simulink model "ar03_sim_RST"  (R2020a)
settings: Solver=ode45  StartTime=0.0  StopTime=38  RelTol=1e-3  EnableMultiTasking=on
values from neighbouring files (symbols this model uses):
  A = [1 0.3 0.2]    [ar03_spustima_RMNS.m]    (also in ar03_spustima_STR.m)
  B = [0 0.15]    [ar03_spustima_RMNS.m]    (also in ar03_spustima_STR.m)
  Tvz = 0.1    [ar03_spustima_RMNS.m]    (also in ar03_spustima_STR.m)
settings Model: Creator=MT  LastModifiedBy=MT
settings DataIOCC: LimitDataPoints=on  SaveFormat=Array  SignalLoggingSaveFormat=ModelDataLogs  SaveOutput=off  SignalLogging=off  SaveTime=off  ReturnWorkspaceOutputs=off
settings OptimizationCC: ExpressionDepthLimit=2147483647  InitFltsAndDblsToZero=on  LifeSpan=inf
settings DebuggingCC: SaveWithParameterizedLinksMsg=none  UnderspecifiedInitializationDetection=Classic  MergeDetectMultiDrivingBlocksExec=none  SignalResolutionControl=TryResolveAllWithWarning  SolverPrmCheckMsg=warning  MultiTaskDSMMsg=warning  MultiTaskCondExecSysMsg=none  FcnCallInpInsideContextMsg=warning  AllowSymbolicDim=off  StateNameClashWarn=warning  SFUnexpectedBacktrackingDiag=warning  SFNoUnconditionalDefaultTransitionDiag=warning  SFExecutionAtInitializationDiag=none  ArithmeticOperatorsInVariantConditions=warning
settings HardwareCC: ProdBitPerPointer=32  ProdBitPerSizeT=32  ProdBitPerPtrDiffT=32  ProdLargestAtomicFloat=None  ProdIntDivRoundTo=Undefined  ProdEndianess=Unspecified  ProdWordSize=32  ProdHWDeviceType=32-bit Generic
settings ModelReferenceCC: PropagateSignalLabelsOutOfModel=off
settings SFSimCC: SimUseLocalCustomCode=off  CustomCodeUndefinedFunction=UseInterfaceOnly
settings RTWCC: RTWUseLocalCustomCode=off
settings CodeAppCC: StateflowObjectComments=on
settings GRTTargetCC: TargetFcnLib=ansi_tfl_tmw.mat  TargetLangStandard=C89/C90 (ANSI)  CombineOutputUpdateFcns=off  GRTInterface=on
settings ConfigComp: CovMetricSettings=dw  CovHtmlReporting=on  CovSaveCumulativeToWorkspaceVar=on  CovSaveSingleToWorkspaceVar=on  CovExternalEMLEnable=off

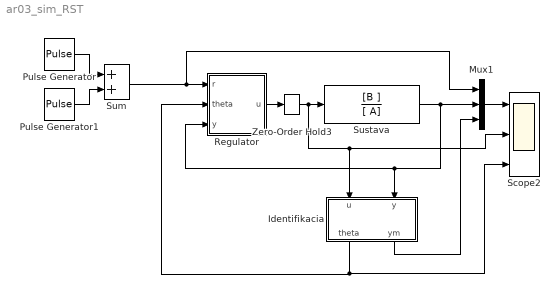
== system ar03_sim_RST ==
  Identifikacia : Subsystem
  Mux1 : Mux  Inputs=3
  Pulse Generator : DiscretePulseGenerator  PulseType=Time based  Period=40  PulseWidth=25
  Pulse Generator1 : DiscretePulseGenerator  PulseType=Time based  Amplitude=-1  Period=40  PulseWidth=25  PhaseDelay=20
  Regulator : Subsystem
  Scope2 : Scope  NumInputPorts=3
  Sum : Sum
  Sustava : TransferFcn  Numerator=[B ]  Denominator=[ A]
  Zero-Order Hold3 : ZeroOrderHold  SampleTime=Tvz
  wires:
  Sustava/1 -> Regulator/3(y), Identifikacia/2(y), Mux1/2
  Identifikacia/1(theta) -> Scope2/3, Regulator/2(theta)
  Mux1/1 -> Scope2/1
  Regulator/1(u) -> Zero-Order Hold3/1
  Zero-Order Hold3/1 -> Scope2/2, Identifikacia/1(u), Sustava/1
  Identifikacia/2(ym) -> Mux1/3
  Pulse Generator/1 -> Sum/1
  Pulse Generator1/1 -> Sum/2
  Sum/1 -> Mux1/1, Regulator/1(r)

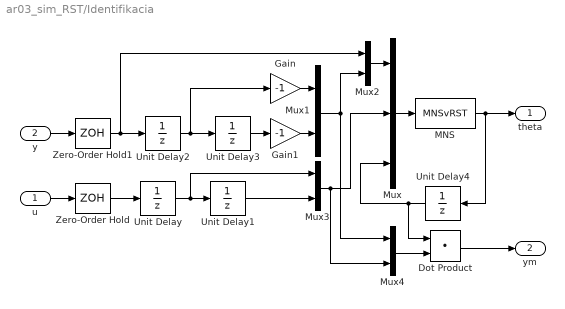
== system ar03_sim_RST/Identifikacia ==
  u : Inport
  y : Inport  Port=2
  Dot Product : DotProduct  InputSameDT=on  OutDataTypeStr=Inherit: Inherit via internal rule
  Gain : Gain  Gain=-1
  Gain1 : Gain  Gain=-1
  MNS : MATLABFcn  MATLABFcn=MNSvRST  OutputDimensions=4
  Mux : Mux  Inputs=3
  Mux{1..4} (4 alike) : Mux  Inputs=2
  Unit Delay{,1..3} (4 alike) : UnitDelay  SampleTime=Tvz  HasFrameUpgradeWarning=on
  Unit Delay4 : UnitDelay  InitialCondition="[-1.5    0.5    -2e-5    1.5e-3]"  SampleTime=Tvz  HasFrameUpgradeWarning=on
  Zero-Order Hold : ZeroOrderHold  SampleTime=Tvz
  Zero-Order Hold1 : ZeroOrderHold  SampleTime=Tvz
  theta : Outport
  ym : Outport  Port=2
  wires:
  u/1 -> Zero-Order Hold/1
  y/1 -> Zero-Order Hold1/1
  Zero-Order Hold/1 -> Unit Delay/1
  Unit Delay/1 -> Unit Delay1/1, Mux3/1
  Zero-Order Hold1/1 -> Unit Delay2/1, Mux2/1
  Unit Delay2/1 -> Unit Delay3/1, Gain/1
  Mux/1 -> MNS/1
  Unit Delay4/1 -> Mux/3, Dot Product/1
  Unit Delay1/1 -> Mux3/2
  Unit Delay3/1 -> Gain1/1
  Gain/1 -> Mux1/1
  Gain1/1 -> Mux1/2
  Mux1/1 -> Mux2/2, Mux4/1
  MNS/1 -> theta/1, Unit Delay4/1
  Dot Product/1 -> ym/1
  Mux2/1 -> Mux/1
  Mux3/1 -> Mux/2, Mux4/2
  Mux4/1 -> Dot Product/2

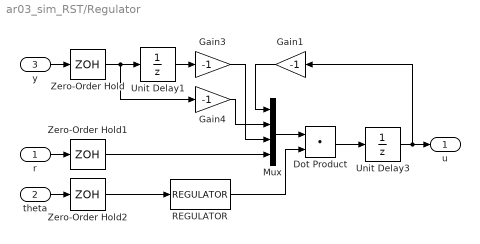
== system ar03_sim_RST/Regulator ==
  r : Inport
  theta : Inport  Port=2
  y : Inport  Port=3
  Dot Product : DotProduct  InputSameDT=on  OutDataTypeStr=Inherit: Inherit via internal rule
  Gain1 : Gain  Gain=-1
  Gain3 : Gain  Gain=-1
  Gain4 : Gain  Gain=-1
  Mux : Mux
  REGULATOR : MATLABFcn  MATLABFcn=REGULATOR  OutputDimensions=4
  Unit Delay1 : UnitDelay  SampleTime=Tvz  HasFrameUpgradeWarning=on
  Unit Delay3 : UnitDelay  SampleTime=Tvz  HasFrameUpgradeWarning=on
  Zero-Order Hold : ZeroOrderHold  SampleTime=Tvz
  Zero-Order Hold1 : ZeroOrderHold  SampleTime=Tvz
  Zero-Order Hold2 : ZeroOrderHold  SampleTime=Tvz
  u : Outport
  wires:
  theta/1 -> Zero-Order Hold2/1
  r/1 -> Zero-Order Hold1/1
  y/1 -> Zero-Order Hold/1
  Zero-Order Hold/1 -> Unit Delay1/1, Gain4/1
  Unit Delay3/1 -> Gain1/1, u/1
  Unit Delay1/1 -> Gain3/1
  Zero-Order Hold2/1 -> REGULATOR/1
  REGULATOR/1 -> Dot Product/2
  Mux/1 -> Dot Product/1
  Gain1/1 -> Mux/1
  Gain3/1 -> Mux/3
  Gain4/1 -> Mux/2
  Zero-Order Hold1/1 -> Mux/4
  Dot Product/1 -> Unit Delay3/1
